simulink model "RateTransitionTut"  (R2024a)
settings: Solver=FixedStepDiscrete  StartTime=0.0  StopTime=10.0  RelTol=1e-3
settings Model: Creator=User  LastModifiedBy=User
settings OptimizationCC: DefaultParameterBehavior=Inlined  EnhancedBackFolding=on  PassReuseOutputArgsAs=Individual arguments  ZeroExternalMemoryAtStartup=off  ZeroInternalMemoryAtStartup=off  OptimizeBlockOrder=speed  DifferentSizesBufferReuse=on  OptimizationCustomize=off  EfficientTunableParamExpr=on
settings DebuggingCC: ParameterTunabilityLossMsg=error
settings SFSimCC: MATLABDynamicMemAlloc=off
settings RTWCC: Description=Embedded Coder  SystemTargetFile=ert.tlc  TemplateMakefile=ert_default_tmf  GenerateReport=on
settings CodeAppCC: ForceParamTrailComments=on  IgnoreCustomStorageClasses=off  OperatorAnnotations=on  SimulinkDataObjDesc=on  SFDataObjDesc=on  InsertBlockDesc=on
settings ERTTargetCC: TargetLangStandard=C99 (ISO)  GenerateSampleERTMain=on  InlinedParameterPlacement=NonHierarchical  ERTCustomFileTemplate=example_file_process.tlc

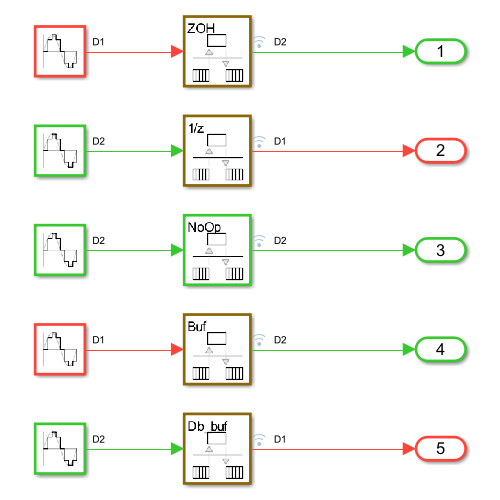
[thumbnail: Simulink's stored preview of the top-level diagram]
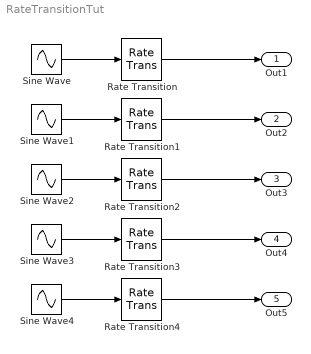
== system RateTransitionTut ==
  Rate Transition : RateTransition
  Rate Transition1 : RateTransition  OutPortSampleTimeOpt=Inherit
  Rate Transition2 : RateTransition
  Rate Transition3 : RateTransition  Deterministic=off
  Rate Transition4 : RateTransition  Deterministic=off  OutPortSampleTimeOpt=Inherit
  Sine Wave : Sin  SampleTime=.1
  Sine Wave1 : Sin  SampleTime=.2
  Sine Wave2 : Sin  SampleTime=.2
  Sine Wave3 : Sin  SampleTime=.1
  Sine Wave4 : Sin  SampleTime=.2
  Out1 : Outport  SampleTime=.2
  Out2 : Outport  Port=2  SampleTime=.1
  Out3 : Outport  Port=3  SampleTime=.2
  Out4 : Outport  Port=4  SampleTime=.2
  Out5 : Outport  Port=5  SampleTime=.1
  wires:
  Sine Wave/1 -> Rate Transition/1
  Rate Transition/1 -> Out1/1
  Rate Transition1/1 -> Out2/1
  Sine Wave1/1 -> Rate Transition1/1
  Sine Wave2/1 -> Rate Transition2/1
  Rate Transition2/1 -> Out3/1
  Rate Transition3/1 -> Out4/1
  Sine Wave3/1 -> Rate Transition3/1
  Sine Wave4/1 -> Rate Transition4/1
  Rate Transition4/1 -> Out5/1
